simulink model "ysw15_9"  (R2014a)
settings: Solver=ode45  StartTime=0.0  StopTime=10.0  RelTol=1e-3
settings Model: Creator=ii  LastModifiedBy=ii
settings SolverCC: ZeroCrossAlgorithm=Adaptive
settings DebuggingCC: UnderspecifiedInitializationDetection=Classic

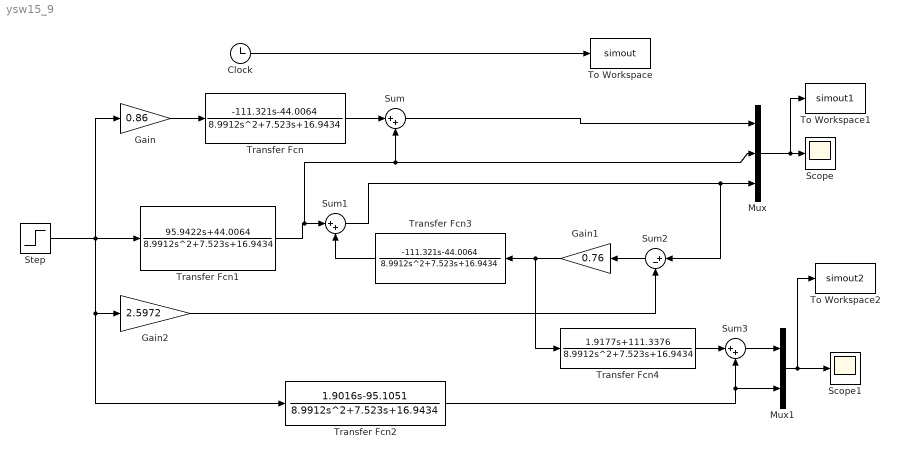
== system ysw15_9 ==
  Clock : Clock
  Gain : Gain  Gain=0.86
  Gain1 : Gain  Gain=0.76
  Gain2 : Gain  Gain=2.5972
  Mux : Mux  Inputs=3
  Mux1 : Mux  Inputs=2
  Scope : Scope
  Scope1 : Scope
  Step : Step  SampleTime=0
  Sum : Sum  Inputs=|++
  Sum1 : Sum  Inputs=|++
  Sum2 : Sum  Inputs=|+-
  Sum3 : Sum  Inputs=|++
  To Workspace : ToWorkspace  VariableName=simout  SampleTime=-1
  To Workspace1 : ToWorkspace  VariableName=simout1  SampleTime=-1
  To Workspace2 : ToWorkspace  VariableName=simout2  SampleTime=-1
  Transfer Fcn : TransferFcn  Numerator=[-111.321,-44.0064]  Denominator=[8.9912 7.523,16.9434]
  Transfer Fcn1 : TransferFcn  Numerator=[95.9422,44.0064]  Denominator=[8.9912 7.523,16.9434]
  Transfer Fcn2 : TransferFcn  Numerator=[1.9016,-95.1051]  Denominator=[8.9912 7.523,16.9434]
  Transfer Fcn3 : TransferFcn  Numerator=[-111.321,-44.0064]  Denominator=[8.9912 7.523,16.9434]
  Transfer Fcn4 : TransferFcn  Numerator=[1.9177,111.3376]  Denominator=[8.9912 7.523,16.9434]
  wires:
  Clock/1 -> To Workspace/1
  Mux/1 -> To Workspace1/1, Scope/1
  Mux1/1 -> To Workspace2/1, Scope1/1
  Gain/1 -> Transfer Fcn/1
  Transfer Fcn/1 -> Sum/1
  Sum/1 -> Mux/1
  Sum3/1 -> Mux1/1
  Step/1 -> Gain/1, Transfer Fcn1/1, Transfer Fcn2/1, Gain2/1
  Transfer Fcn2/1 -> Sum3/2, Mux1/2
  Transfer Fcn1/1 -> Sum/2, Mux/2, Sum1/1
  Sum1/1 -> Sum2/1, Mux/3
  Sum2/1 -> Gain1/1
  Gain1/1 -> Transfer Fcn3/1, Transfer Fcn4/1
  Transfer Fcn3/1 -> Sum1/2
  Gain2/1 -> Sum2/2
  Transfer Fcn4/1 -> Sum3/1
